simulink model "te_plant_controller_for_omnet"  (R2013b)
settings: Solver=ode5  SolverMode=SingleTasking  StartTime=0.0044444  StopTime=0.0047222  FixedStep=Ts_base  MaxStep=Ts_base  MinStep=1e-6  RelTol=1e-6
InitFcn:
  | %global model_type
  | %model_type = 0
  | 
  | %init_model
StopFcn:
  | %TEplot
values from neighbouring files (symbols this model uses):
  Ts_base = (10e-3)/3600    (= 2.77777777778e-06)    [init_model_omnet.m]    (also in run_tesim_init.m = 0.000277777777778; run_tesim_next.m = 0.000277777777778)
  Ts_save = 1/3600    (= 0.000277777777778)    [init_model_omnet.m]    (also in run_tesim_init.m; run_tesim_next.m)
  xmeas_in = xmeas_out    [run_tesim_func.m]    (also in run_tesim_init.m = dlmread('xmeas_in.txt', '\t'); run_tesim_next.m = dlmread('xmeas_in.txt'))
  xmv_in = xmv_out    [run_tesim_func.m]    (also in run_tesim_init.m = u0([1 2 3 4 6 7 8 10 11]); run_tesim_next.m = dlmread('xmv_in.txt'))
libraries: TEsim_utils x2
settings Model: Creator=rnc4  LastModifiedBy=rnc4
settings DataIOCC: LimitDataPoints=off  LoadInitialState=on  SaveFinalState=on  SaveFormat=Structure  SignalLoggingSaveFormat=ModelDataLogs  ReturnWorkspaceOutputs=on  SignalLoggingName=sigsOut
settings OptimizationCC: InitFltsAndDblsToZero=on
settings DebuggingCC: SaveWithParameterizedLinksMsg=none  SignalResolutionControl=TryResolveAllWithWarning  SolverPrmCheckMsg=none  MultiTaskDSMMsg=warning  MultiTaskCondExecSysMsg=none  FcnCallInpInsideContextMsg=UseLocalSettings  SimStateOlderReleaseMsg=warning
settings HardwareCC: TargetUnknown=on
settings RTWCC: IncludeERTFirstTime=on
settings GRTTargetCC: TargetFcnLib=ansi_tfl_tmw.mat  CodeReplacementLibrary=None  CombineOutputUpdateFcns=off  CPPClassGenCompliant=on  GRTInterface=on

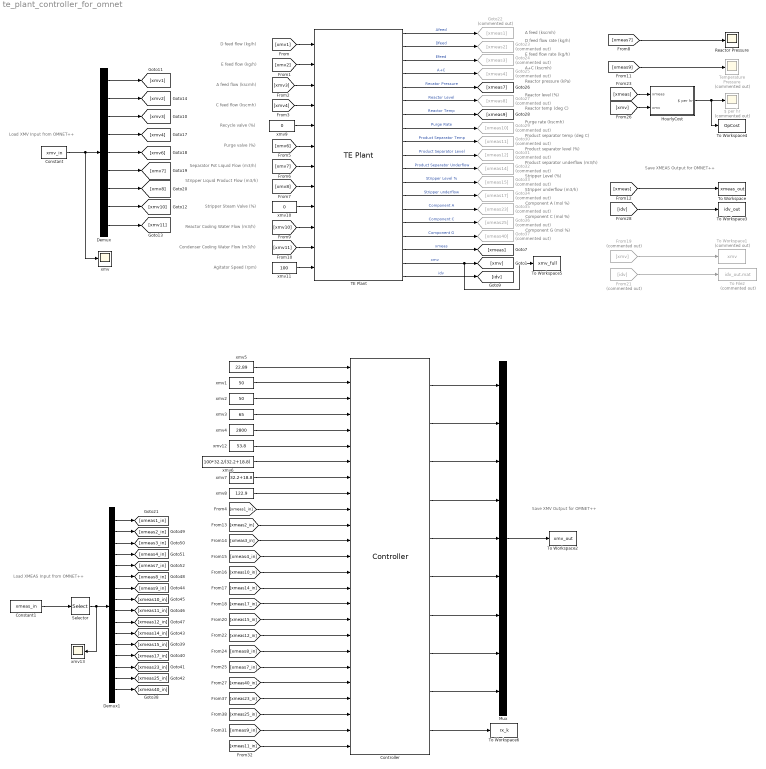
== system te_plant_controller_for_omnet ==
  note: Agitator Speed (rpm)
  note: Condenser Cooling Water Flow (m3/h)
  note: Reactor Cooling Water Flow (m3/h)
  note: Stripper Steam Valve (%)
  note: Stripper Liquid Product Flow (m3/h)
  note: Separator Pot Liquid Flow (m3/h)
  note: Purge valve (%)
  note: Recycle valve (%)
  note: C feed flow (kscmh)
  note: A feed flow (kscmh)
  note: E feed flow (kg/h)
  note: D feed flow (kg/h)
  note: Component G (mol %)
  note: Component C (mol %)
  note: Component A (mol %)
  note: Stripper underflow (m3/h)
  note: Stripper Level (%)
  note: Product separator underflow (m3/h)
  note: Product separator level (%)
  note: Product separator temp (deg C)
  note: Purge rate (kscmh)
  note: Reactor temp (deg C)
  note: Reactor level (%)
  note: Reactor pressure (kPa)
  note: A+C (kscmh)
  note: E feed flow rate (kg/h)
  note: D feed flow rate (kg/h)
  note: A feed (kscmh)
  note: Save XMV Output for OMNET++
  note: Load XMV Input from OMNET++
  note: Save XMEAS Output for OMNET++
  note: Load XMEAS Input from OMNET++
  $ per hr : Scope  Commented=on
      settings: YMin=75  YMax=400  SaveName=OpCost  SampleInput=on  SampleTime=Ts_save
  Constant : Constant  Value=xmv_in  SampleTime=Ts_base
  Constant1 : Constant  Value=xmeas_in  SampleTime=Ts_base
  Controller : TEsim_utils/TEsim/Controller
  Demux : Demux  Outputs=9
  Demux1 : Demux  Outputs=16
  From19 : From  Commented=on  GotoTag=xmv
      settings: CloseFcn=tagdialog Close
  From21 : From  Commented=on  GotoTag=idv
      settings: CloseFcn=tagdialog Close
  Goto22 : Goto  Commented=on  GotoTag=xmeas1
  Goto23 : Goto  Commented=on  GotoTag=xmeas2
  Goto24 : Goto  Commented=on  GotoTag=xmeas3
  Goto25 : Goto  Commented=on  GotoTag=xmeas4
  Goto27 : Goto  Commented=on  GotoTag=xmeas8
  Goto29 : Goto  Commented=on  GotoTag=xmeas10
  Goto30 : Goto  Commented=on  GotoTag=xmeas11
  Goto31 : Goto  Commented=on  GotoTag=xmeas12
  Goto32 : Goto  Commented=on  GotoTag=xmeas14
  Goto33 : Goto  Commented=on  GotoTag=xmeas15
  Goto34 : Goto  Commented=on  GotoTag=xmeas17
  Goto35 : Goto  Commented=on  GotoTag=xmeas23
  Goto36 : Goto  Commented=on  GotoTag=xmeas25
  Goto37 : Goto  Commented=on  GotoTag=xmeas40
  HourlyCost : Subsystem
  Mux : Mux  Inputs=9
  Reactor Pressure : Scope
      settings: TimeRange=0.0003  YMin=2704.75  YMax=2705  SampleInput=on  SampleTime=Ts_save
  Selector : Selector  InputPortWidth=41  IndexOptions=Index vector (dialog)  Indices=[1:4, 7:12, 14, 15, 17, 23, 25, 40]  OutputSizes=1
  TE Plant : TEsim_utils/TEsim/TE Plant  tesim_ic=tesim_ic
  Temperature Pressure : Scope  Commented=on
      settings: TimeRange=15  YMin=122.85  YMax=122.95  SampleInput=on  SampleTime=Ts_save
  To File2 : ToFile  Commented=on  Filename=idv_out.mat  MatrixName=idv_out
  To Workspace : ToWorkspace  VariableName=xmeas_out  SampleTime=Ts_base
      settings: MaxDataPoints=1
  To Workspace1 : ToWorkspace  Commented=on  VariableName=xmv  SampleTime=Ts_save
  To Workspace2 : ToWorkspace  VariableName=xmv_out  SampleTime=Ts_base
      settings: MaxDataPoints=1
  To Workspace3 : ToWorkspace  VariableName=idv_out  SampleTime=Ts_base
      settings: MaxDataPoints=1
  To Workspace4 : ToWorkspace  VariableName=OpCost  SampleTime=Ts_save
  To Workspace5 : ToWorkspace  VariableName=xmv_full  SampleTime=Ts_base
      settings: MaxDataPoints=1
  To Workspace6 : ToWorkspace  VariableName=rx_k  SampleTime=Ts_base
      settings: MaxDataPoints=1
  xmv : Scope
      settings: TimeRange=0.0003  YMin=2704.75  YMax=2705  SaveName=ScopeData2  SampleInput=on  SampleTime=Ts_save
  xmv1 : Constant  Value=50
  xmv10 : Constant  Value=0
  xmv11 : Constant  Value=100
  xmv12 : Constant  Value=53.8
  xmv13 : Scope
      settings: TimeRange=0.0003  YMin=2704.75  YMax=2705  SaveName=ScopeData3  SampleInput=on  SampleTime=Ts_save
  xmv2 : Constant  Value=50
  xmv3 : Constant  Value=65
  xmv4 : Constant  Value=2800
  xmv5 : Constant  Value=22.89
  xmv6 : Constant  Value=100*32.2/(32.2+18.8)
  xmv7 : Constant  Value=32.2+18.8
  xmv8 : Constant  Value=122.9
  xmv9 : Constant  Value=0
  wires:
  HourlyCost/1($ per hr) -> To Workspace4/1, $ per hr/1
  xmv8/1 -> Controller/9
  xmv7/1 -> Controller/8
  xmv6/1 -> Controller/7
  xmv12/1 -> Controller/6
  xmv4/1 -> Controller/5
  xmv3/1 -> Controller/4
  xmv2/1 -> Controller/3
  xmv1/1 -> Controller/2
  xmv5/1 -> Controller/1
  TE Plant/7 -> [xmeas9]  "Reactor Temp"
  TE Plant/5 -> [xmeas7]  "Recator Pressure"
  TE Plant/18 -> To Workspace5/1, [xmv]  "xmv"
  TE Plant/17 -> [xmeas]  "xmeas"
  [xmv1] -> TE Plant/1
  [xmv2] -> TE Plant/2
  [xmv3] -> TE Plant/3
  [xmv4] -> TE Plant/4
  xmv9/1 -> TE Plant/5
  [xmv6] -> TE Plant/6
  [xmv7] -> TE Plant/7
  [xmv8] -> TE Plant/8
  xmv10/1 -> TE Plant/9
  [xmv10] -> TE Plant/10
  [xmv11] -> TE Plant/11
  xmv11/1 -> TE Plant/12
  TE Plant/1 -> Goto22/1  "Afeed"
  TE Plant/2 -> Goto23/1  "Dfeed"
  TE Plant/3 -> Goto24/1  "Efeed"
  TE Plant/4 -> Goto25/1  "A+C"
  TE Plant/6 -> Goto27/1  "Reactor Level"
  TE Plant/8 -> Goto29/1  "Purge Rate"
  TE Plant/9 -> Goto30/1  "Product Separator Temp"
  TE Plant/10 -> Goto31/1  "Product Separator Level"
  TE Plant/11 -> Goto32/1  "Product Separator Underflow"
  TE Plant/12 -> Goto33/1  "Stripper Level %"
  TE Plant/13 -> Goto34/1  "Stripper underflow"
  TE Plant/14 -> Goto35/1  "Component A"
  TE Plant/15 -> Goto36/1  "Component C"
  TE Plant/16 -> Goto37/1  "Component G"
  TE Plant/19 -> [idv]  "idv"
  [xmeas7] -> Reactor Pressure/1
  [xmeas9] -> Temperature Pressure/1
  [xmeas] -> To Workspace/1
  From19/1 -> To Workspace1/1
  From21/1 -> To File2/1
  [xmeas] -> HourlyCost/1(xmeas)
  [xmv] -> HourlyCost/2(xmv)
  Mux/1 -> To Workspace2/1
  Demux/1 -> [xmv1]
  Demux/2 -> [xmv2]
  Demux/3 -> [xmv3]
  Demux/4 -> [xmv4]
  Demux/5 -> [xmv6]
  Demux/6 -> [xmv7]
  Demux/7 -> [xmv8]
  Demux/8 -> [xmv10]
  Demux/9 -> [xmv11]
  Demux1/1 -> [xmeas1_in]
  Demux1/2 -> [xmeas2_in]
  Demux1/3 -> [xmeas3_in]
  Demux1/4 -> [xmeas4_in]
  Demux1/5 -> [xmeas7_in]
  Demux1/6 -> [xmeas8_in]
  Demux1/7 -> [xmeas9_in]
  Demux1/8 -> [xmeas10_in]
  Demux1/9 -> [xmeas11_in]
  Demux1/10 -> [xmeas12_in]
  Demux1/11 -> [xmeas14_in]
  Demux1/12 -> [xmeas15_in]
  Demux1/13 -> [xmeas17_in]
  Demux1/14 -> [xmeas23_in]
  Demux1/15 -> [xmeas25_in]
  Demux1/16 -> [xmeas40_in]
  Selector/1 -> xmv13/1, Demux1/1
  Controller/5 -> Mux/5
  Controller/4 -> Mux/4
  Controller/6 -> Mux/6
  Controller/3 -> Mux/3
  Controller/7 -> Mux/7
  Controller/2 -> Mux/2
  Controller/8 -> Mux/8
  Controller/1 -> Mux/1
  Controller/9 -> Mux/9
  [xmeas4_in] -> Controller/13
  [xmeas10_in] -> Controller/14
  [xmeas14_in] -> Controller/15
  [xmeas17_in] -> Controller/16
  [xmeas15_in] -> Controller/17
  [xmeas12_in] -> Controller/18
  [xmeas8_in] -> Controller/19
  [xmeas7_in] -> Controller/20
  [xmeas40_in] -> Controller/21
  [xmeas9_in] -> Controller/24
  [xmeas11_in] -> Controller/25
  [xmeas23_in] -> Controller/22
  [xmeas25_in] -> Controller/23
  [xmeas2_in] -> Controller/11
  [xmeas3_in] -> Controller/12
  [xmeas1_in] -> Controller/10
  [idv] -> To Workspace3/1
  Constant/1 -> xmv/1, Demux/1
  Controller/10 -> To Workspace6/1
  Constant1/1 -> Selector/1

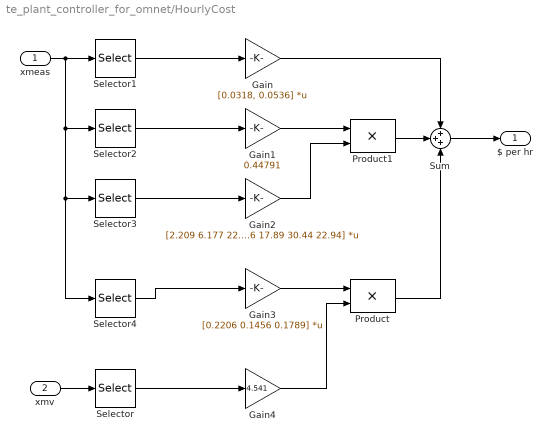
== system te_plant_controller_for_omnet/HourlyCost ==
  xmeas : Inport  PortDimensions=41
  xmv : Inport  Port=2  PortDimensions=12
  Gain : Gain  Gain=[0.0318, 0.0536]  Multiplication=Matrix(K*u)  SaturateOnIntegerOverflow=on  OutDataTypeStr=Inherit: Same as input  ParamDataTypeStr=Inherit: Same as input
      settings: AttributesFormatString=%<Gain>
  Gain1 : Gain  Gain=0.44791  SaturateOnIntegerOverflow=on  OutDataTypeStr=Inherit: Same as input  ParamDataTypeStr=Inherit: Same as input
      settings: AttributesFormatString=%<Gain>
  Gain2 : Gain  Gain=[2.209 6.177 22.06 14.56 17.89 30.44 22.94]  Multiplication=Matrix(K*u)  SaturateOnIntegerOverflow=on  OutDataTypeStr=Inherit: Same as input  ParamDataTypeStr=Inherit: Same as input
      settings: AttributesFormatString=%<Gain>
  Gain3 : Gain  Gain=[0.2206 0.1456 0.1789]  Multiplication=Matrix(K*u)  SaturateOnIntegerOverflow=on  OutDataTypeStr=Inherit: Same as input  ParamDataTypeStr=Inherit: Same as input
      settings: AttributesFormatString=%<Gain>
  Gain4 : Gain  Gain=4.541  SaturateOnIntegerOverflow=on  OutDataTypeStr=Inherit: Same as input  ParamDataTypeStr=Inherit: Same as input
      settings: AttributesFormatString=%<Gain>
  Product : Product  SaturateOnIntegerOverflow=on  OutDataTypeStr=Inherit: Same as first input
  Product1 : Product  SaturateOnIntegerOverflow=on  OutDataTypeStr=Inherit: Same as first input
  Selector : Selector  InputPortWidth=12  IndexOptions=Index vector (dialog)  Indices=8  OutputSizes=1
  Selector1 : Selector  InputPortWidth=41  IndexOptions=Index vector (dialog)  Indices=[19 20]  OutputSizes=1
  Selector2 : Selector  InputPortWidth=41  IndexOptions=Index vector (dialog)  Indices=[10]  OutputSizes=1
  Selector3 : Selector  InputPortWidth=41  IndexOptions=Index vector (dialog)  Indices=[29, 31:36]  OutputSizes=1
  Selector4 : Selector  InputPortWidth=41  IndexOptions=Index vector (dialog)  Indices=[37:39]  OutputSizes=1
  Sum : Sum  Inputs=+++  SaturateOnIntegerOverflow=on
  $ per hr : Outport
  wires:
  xmv/1 -> Selector/1
  xmeas/1 -> Selector1/1, Selector2/1, Selector3/1, Selector4/1
  Selector1/1 -> Gain/1
  Selector2/1 -> Gain1/1
  Selector3/1 -> Gain2/1
  Selector4/1 -> Gain3/1
  Selector/1 -> Gain4/1
  Gain3/1 -> Product/1
  Gain4/1 -> Product/2
  Sum/1 -> $ per hr/1
  Product/1 -> Sum/3
  Gain/1 -> Sum/1
  Product1/1 -> Sum/2
  Gain1/1 -> Product1/1
  Gain2/1 -> Product1/2
